simulink library "csu_gtb_gravity_three_body_moon_lib"  (R2014b)
settings: Solver=ode45  SolverMode=SingleTasking  StartTime=0.0  StopTime=10.0  RelTol=1e-3
libraries: util_info_lib x1, csu_grv_gravity_model_lib x1, csu_eph_spice_lib x1
settings Model: ExtModeAutoUpdateStatusClock=off  Creator=daniloviazzo  LastModifiedBy=mstewart

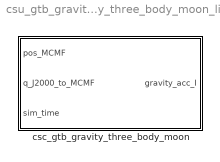
== system csu_gtb_gravity_three_body_moon_lib ==
  csc_gtb_gravity_three_body_moon : Subsystem

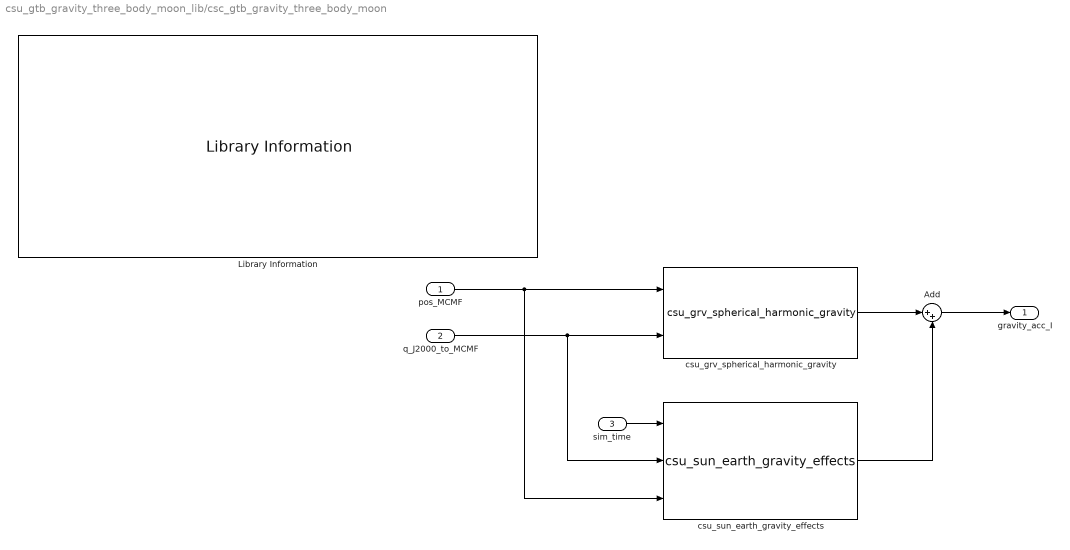
== system csu_gtb_gravity_three_body_moon_lib/csc_gtb_gravity_three_body_moon ==
  pos_MCMF : Inport
  q_J2000_to_MCMF : Inport  Port=2
  sim_time : Inport  Port=3
  Add : Sum  Inputs=|++
  Library Information : util_info_lib/Library Information  owner='NONE'
  csu_grv_spherical_harmonic_gravity : csu_grv_gravity_model_lib/csu_grv_spherical_harmonic_gravity
  csu_sun_earth_gravity_effects : csu_eph_spice_lib/csu_sun_earth_gravity_effects
  gravity_acc_I : Outport
  wires:
  pos_MCMF/1 -> csu_sun_earth_gravity_effects/3, csu_grv_spherical_harmonic_gravity/1
  q_J2000_to_MCMF/1 -> csu_sun_earth_gravity_effects/2, csu_grv_spherical_harmonic_gravity/2
  sim_time/1 -> csu_sun_earth_gravity_effects/1
  csu_sun_earth_gravity_effects/1 -> Add/2
  csu_grv_spherical_harmonic_gravity/1 -> Add/1
  Add/1 -> gravity_acc_I/1
